simulink library "stateEquations_ul"  (R2018b)
settings: Solver=VariableStepAuto  StartTime=0.0  StopTime=10.0  RelTol=1e-3
undefined symbols (not defined in the file): headingTimeConstant_s, maxSteadySpeed_mPs, speedTimeConstant_s
settings Model: Creator=mcobb  LastModifiedBy=mcobb
settings DebuggingCC: LibraryContextMissingDiagnostic=none
settings SFSimCC: SimUseLocalCustomCode=off
settings RTWCC: RTWUseLocalCustomCode=off

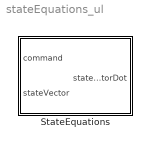
== system stateEquations_ul ==
  StateEquations : Subsystem

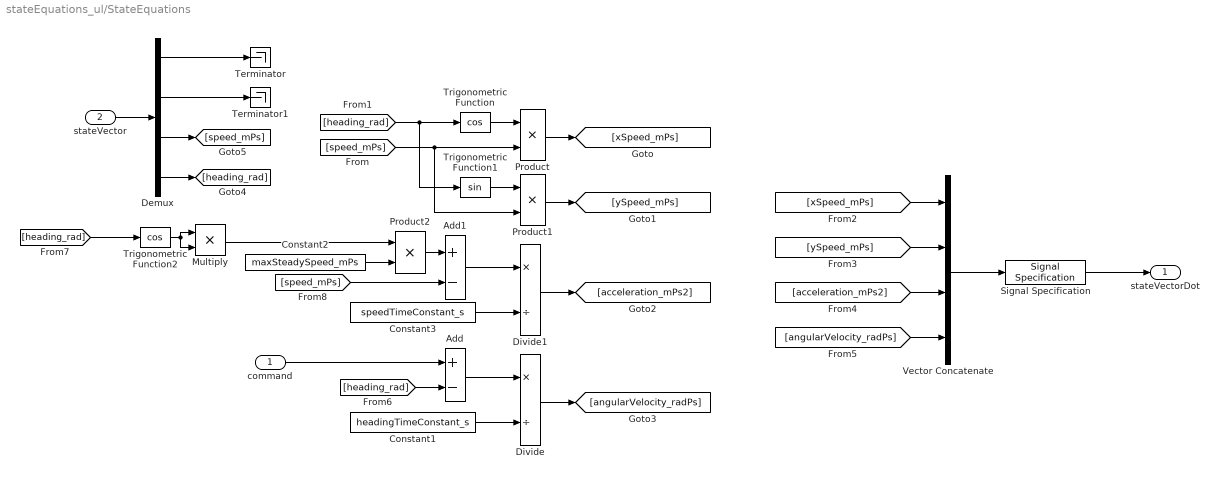
== system stateEquations_ul/StateEquations ==
  command : Inport
  stateVector : Inport  Port=2
  Add : Sum  Inputs=+-
  Add1 : Sum  Inputs=+-
  Constant1 : Constant  Value=headingTimeConstant_s
  Constant2 : Constant  Value=maxSteadySpeed_mPs
  Constant3 : Constant  Value=speedTimeConstant_s
  Demux : Demux
  Divide : Product  Inputs=*/
  Divide1 : Product  Inputs=*/
  Multiply : Product
  Product : Product
  Product1 : Product
  Product2 : Product
  Signal Specification : SignalSpecification  Dimensions=[4 1]
  Terminator : Terminator
  Terminator1 : Terminator
  Trigonometric Function : Trigonometry  Operator=cos
  Trigonometric Function1 : Trigonometry
  Trigonometric Function2 : Trigonometry  Operator=cos
  Vector Concatenate : Concatenate  NumInputs=4
  stateVectorDot : Outport
  wires:
  [heading_rad] -> Add/2
  Product2/1 -> Add1/1
  Product1/1 -> [ySpeed_mPs]
  Demux/4 -> [heading_rad]
  Trigonometric Function2/1 -> Multiply/2, Multiply/1
  command/1 -> Add/1
  [angularVelocity_radPs] -> Vector Concatenate/4
  Divide/1 -> [angularVelocity_radPs]
  [ySpeed_mPs] -> Vector Concatenate/2
  stateVector/1 -> Demux/1
  Vector Concatenate/1 -> Signal Specification/1
  Product/1 -> [xSpeed_mPs]
  Demux/1 -> Terminator/1
  Signal Specification/1 -> stateVectorDot/1
  [heading_rad] -> Trigonometric Function2/1
  Demux/3 -> [speed_mPs]
  [acceleration_mPs2] -> Vector Concatenate/3
  Multiply/1 -> Product2/1
  [speed_mPs] -> Add1/2
  Trigonometric Function/1 -> Product/1
  Constant3/1 -> Divide1/2
  Add/1 -> Divide/1
  Add1/1 -> Divide1/1
  [xSpeed_mPs] -> Vector Concatenate/1
  Demux/2 -> Terminator1/1
  [speed_mPs] -> Product/2, Product1/2
  Trigonometric Function1/1 -> Product1/1
  [heading_rad] -> Trigonometric Function1/1, Trigonometric Function/1
  Divide1/1 -> [acceleration_mPs2]
  Constant1/1 -> Divide/2
  Constant2/1 -> Product2/2
